simulink model "test_led_on"  (R2023b)
settings: Solver=VariableStepAuto  StartTime=0.0  StopTime=60  RelTol=1e-3
settings Model: Creator=Asus  LastModifiedBy=Asus
settings OptimizationCC: ReuseModelBlockBuffer=off

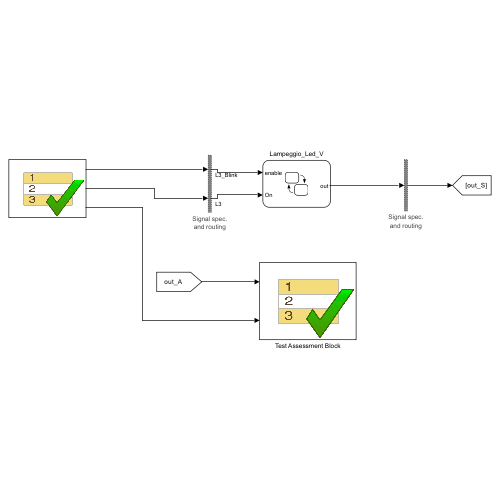
[thumbnail: Simulink's stored preview of the top-level diagram]
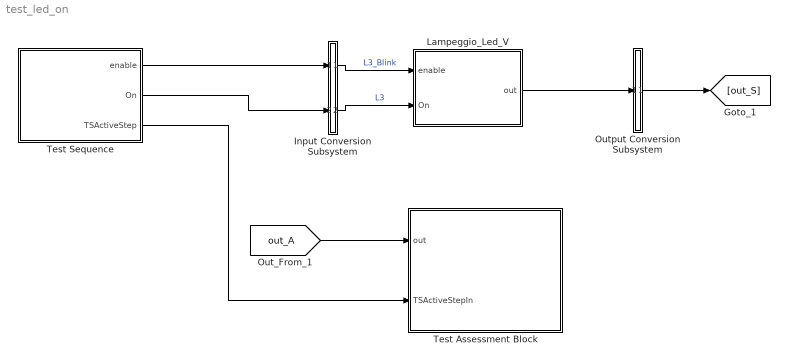
== system test_led_on ==
  Input Conversion Subsystem : Subsystem  Tag=__SLT_ICS__  Description=|
      | Signal spec.
      | and routing
      settings: AttributesFormatString=%<Description>
  Lampeggio_Led_V : Stateflow chart  TreatAsAtomicUnit=on
  Output Conversion Subsystem : Subsystem  Tag=__SLT_OCS__  Description=|
      | Signal spec.
      | and routing
      settings: AttributesFormatString=%<Description>
  Test Assessment Block : Test Sequence  Tag=__SLT_ASMT__  TreatAsAtomicUnit=on
  Test Sequence : Test Sequence  TreatAsAtomicUnit=on
  wires:
  [out_A] -> Test Assessment Block/1(out)
  Test Sequence/1(enable) -> Input Conversion Subsystem/1(Inport_1)
  Test Sequence/2(On) -> Input Conversion Subsystem/2(Inport_2)
  Output Conversion Subsystem/1(Outport_1) -> [out_S]
  Input Conversion Subsystem/1(Outport_1) -> Lampeggio_Led_V/1(enable)  "L3_Blink"
  Input Conversion Subsystem/2(Outport_2) -> Lampeggio_Led_V/2(On)  "L3"
  Lampeggio_Led_V/1(out) -> Output Conversion Subsystem/1(Inport_1)
  Test Sequence/3(TSActiveStep) -> Test Assessment Block/2(TSActiveStepIn)

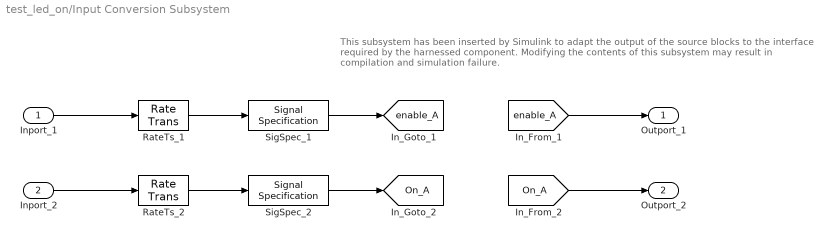
== system test_led_on/Input Conversion Subsystem ==
  note: This subsystem has been inserted by Simulink to adapt the output of the source blocks to the interface required by the harnessed component.
      |  Modifying the contents of this subsystem may result in compilation and simulation failure.
  Inport_1 : Inport
  Inport_2 : Inport  Port=2
  RateTs_1 : RateTransition  OutPortSampleTime=[0, 1]
  RateTs_2 : RateTransition  OutPortSampleTime=[0, 1]
  SigSpec_1 : SignalSpecification  OutDataTypeStr=boolean  Dimensions=[1]  SampleTime=[0, 1]
  SigSpec_2 : SignalSpecification  OutDataTypeStr=boolean  Dimensions=[1]  SampleTime=[0, 1]
  Outport_1 : Outport
  Outport_2 : Outport  Port=2
  tag scope: On_A=global, enable_A=global
  wires:
  [enable_A] -> Outport_1/1
  SigSpec_1/1 -> [enable_A]
  RateTs_1/1 -> SigSpec_1/1
  Inport_1/1 -> RateTs_1/1
  [On_A] -> Outport_2/1
  SigSpec_2/1 -> [On_A]
  RateTs_2/1 -> SigSpec_2/1
  Inport_2/1 -> RateTs_2/1

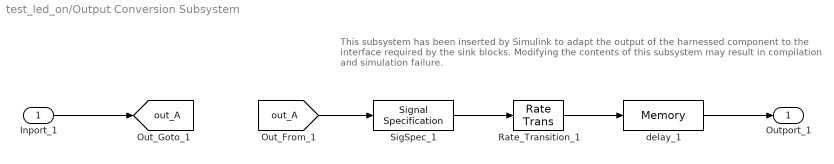
== system test_led_on/Output Conversion Subsystem ==
  note: This subsystem has been inserted by Simulink to adapt the output of the harnessed component to the interface required by the sink blocks.
      |  Modifying the contents of this subsystem may result in compilation and simulation failure.
  Inport_1 : Inport
  Rate_Transition_1 : RateTransition  OutPortSampleTimeOpt=Inherit
  SigSpec_1 : SignalSpecification  OutDataTypeStr=boolean  Dimensions=[1]
  delay_1 : Memory
  Outport_1 : Outport
  tag scope: out_A=global
  wires:
  Inport_1/1 -> [out_A]
  [out_A] -> SigSpec_1/1
  SigSpec_1/1 -> Rate_Transition_1/1
  Rate_Transition_1/1 -> delay_1/1
  delay_1/1 -> Outport_1/1

== stateflow chart test_led_on/Test Sequence ==
  settings: sampleTime=2.4
  state Init
    %% Initialize data outputs.
    On = false;
    enable;
    settings: description=Situazione iniziale in cui il led è spento
  state LedActive
    On = true;
    settings: description=|
        | Viene richiesta l'accensione del led il quale rimane acceso finche On=true.
        | Mi fermo in questo step per 10 secondi (valore messo di prova)
  state Stop
    On = false;
    settings: description=|
        | Potrei evitare questo step tornando allo stato iniziale.
        | Il lampeggio con enable è gestito in test_led_enable
  (default) -> Init
  Init -> LedActive : [
      | true
      | ]
  LedActive -> Stop : [
      | after(10,sec)
      | ]
  data: enable output boolean size=[1]; On output boolean size=[1]; TSActiveStep output Enum: TSActiveStepEnumH1

== stateflow chart test_led_on/Lampeggio_Led_V ==
  state blink
    state blink_on
      en: out = ACTIVE
    state blink_off
      en: out = DISACTIVE
    (default) -> blink_on
    blink_off -> blink_on : after(period, msec)
    blink_on -> blink_off : after(period, msec)
  state off
    en: out = DISACTIVE;
  state on
    en:out = ACTIVE
  (default) -> off
  off -> blink [order 1] : [enable == ACTIVE]
  off -> on [order 2] : [On==ACTIVE]
  blink -> off : [enable == DISACTIVE]
  on -> off : [On == DISACTIVE]
  data: enable input boolean; out output boolean; ACTIVE constant boolean =true; DISACTIVE constant boolean =false; period constant double =1000; On input boolean

== stateflow chart test_led_on/Test Assessment Block ==
  state Run
    state VerifyInit
      verify(~out)
    state VerifyLedActive
      verify(out)
    state VerifyStop
      verify(~out)
    state Run_1
    (default) -> (junction 22)
    Run -> (junction 22)
    (junction 22) -> (junction 23) [order 1] : [TSActiveStepIn==TSActiveStepEnumH1.Init
        | ]
    (junction 23) -> VerifyInit [order 1] : [~in(Run.VerifyInit)]
    (junction 22) -> (junction 31) [order 2]
    (junction 23) -> (junction 26) [order 2]
    (junction 31) -> (junction 32) [order 1] : [TSActiveStepIn==TSActiveStepEnumH1.LedActive
        | ]
    (junction 32) -> VerifyLedActive [order 1] : [~in(Run.VerifyLedActive)]
    (junction 31) -> (junction 43) [order 2]
    (junction 32) -> (junction 35) [order 2]
    (junction 43) -> (junction 44) [order 1] : [TSActiveStepIn==TSActiveStepEnumH1.Stop
        | ]
    (junction 44) -> VerifyStop [order 1] : [~in(Run.VerifyStop)]
    (junction 43) -> (junction 51) [order 2]
    (junction 44) -> (junction 47) [order 2]
    (junction 51) -> (junction 52)
    (junction 52) -> Run_1 [order 1] : [~in(Run.Run_1)]
    (junction 52) -> (junction 55) [order 2]
  (default) -> Run
  data: out input boolean size=[1]; TSActiveStepIn input
